simulink model "problem7"  (R2022a)
settings: Solver=VariableStepAuto  StartTime=0.0  StopTime=5  RelTol=1e-3
settings Model: Creator=prafu  LastModifiedBy=prafu

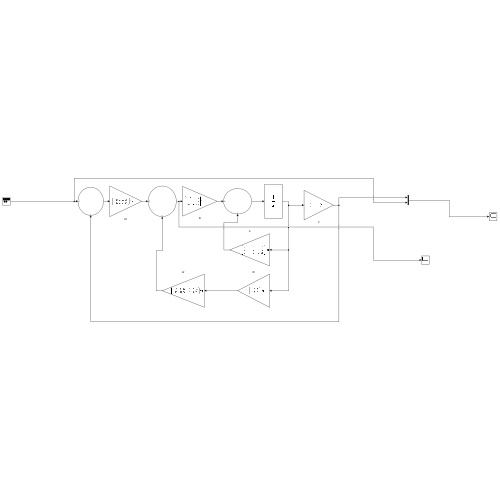
[thumbnail: Simulink's stored preview of the top-level diagram]
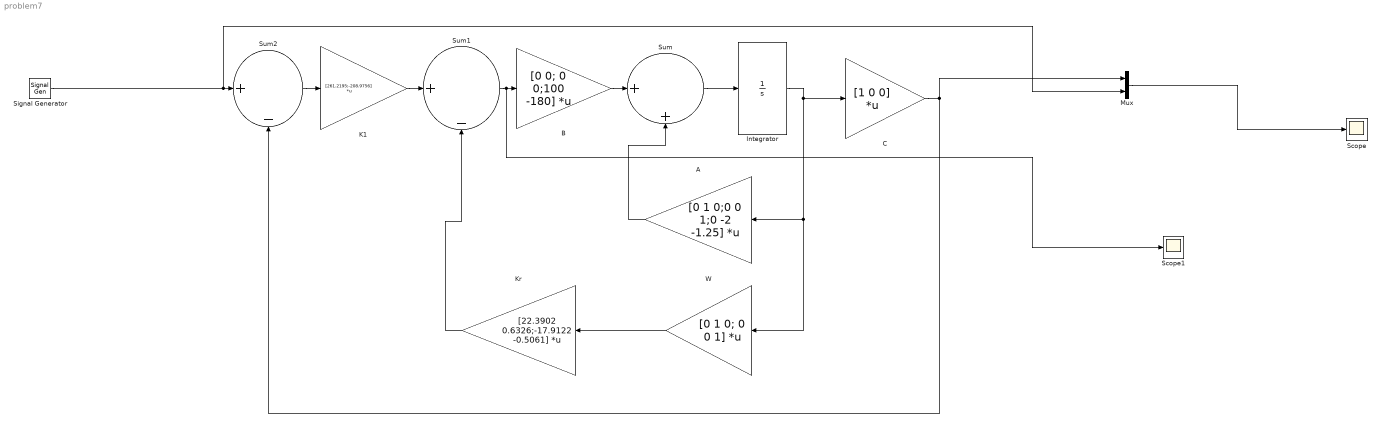
== system problem7 ==
  A : Gain  Gain=[0 1 0;0 0 1;0 -2 -1.25]  Multiplication=Matrix(K*u)
  B : Gain  Gain=[0 0; 0 0;100 -180]  Multiplication=Matrix(K*u)
  C : Gain  Gain=[1 0 0]  Multiplication=Matrix(K*u)
  Integrator : Integrator  InitialCondition=[1;0;0]
  K1 : Gain  Gain=[261.2195;-208.9756]  Multiplication=Matrix(K*u)
  Kr : Gain  Gain=[22.3902 0.6326;-17.9122 -0.5061]  Multiplication=Matrix(K*u)
  Mux : Mux  Inputs=2
  Scope : Scope
  Scope1 : Scope
  Signal Generator : SignalGenerator  WaveForm=square  Frequency=5  Units=rad/sec  VectorParams1D=off
  Sum : Sum  Inputs=|++
  Sum1 : Sum  Inputs=|+-
  Sum2 : Sum  Inputs=|+-
  W : Gain  Gain=[0 1 0; 0 0 1]  Multiplication=Matrix(K*u)
  wires:
  Sum1/1 -> Scope1/1, B/1
  A/1 -> Sum/2
  Integrator/1 -> C/1, W/1, A/1
  Sum/1 -> Integrator/1
  B/1 -> Sum/1
  W/1 -> Kr/1
  Kr/1 -> Sum1/2
  K1/1 -> Sum1/1
  C/1 -> Mux/1, Sum2/2
  Sum2/1 -> K1/1
  Signal Generator/1 -> Mux/2, Sum2/1
  Mux/1 -> Scope/1
